simulink model "Tanques"  (R2020a)
settings: Solver=VariableStepAuto  StartTime=0.0  StopTime=10.0  RelTol=1e-3
settings Model: Creator=Miguel Gutierrez  LastModifiedBy=Miguel Gutierrez

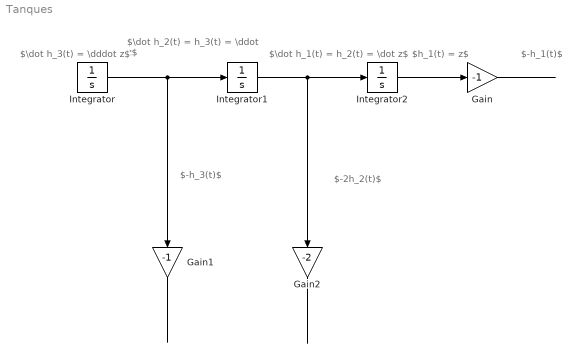
== system Tanques ==
  note: $-h_1(t)$
  note: $\dot h_1(t) = h_2(t) = \dot z$
  note: $\dot h_2(t) = h_3(t) = \ddot z$
  note: $\dot h_3(t) = \dddot z$
  note: $h_1(t) = z$
  note: $-h_3(t)$
  note: $-2h_2(t)$
  Gain : Gain  Gain=-1
  Gain1 : Gain  Gain=-1
  Gain2 : Gain  Gain=-2
  Integrator : Integrator
  Integrator1 : Integrator
  Integrator2 : Integrator
  wires:
  ? -> Integrator/1
  Integrator/1 -> Gain1/1, Integrator1/1
  Integrator1/1 -> Integrator2/1, Gain2/1
  Integrator2/1 -> Gain/1
  Gain/1 -> ?
  Gain1/1 -> ?
  Gain2/1 -> ?
